simulink model "gm_DVBS"  (R2023b)
settings: Solver=FixedStepAuto  StartTime=0.0  StopTime=160000/fs  FixedStep=5e-9  RelTol=1e-3  EnableMultiTasking=on
undefined symbols (not defined in the file or in its folder): ctrlIn, fc, fs, iniStates, k, n, oneData, rb, Rcos, simDataIn, sourceData
libraries: simulink x29, hdlsllib x23, commdigbbndpm3 x4, commhdlblkcod x4, dspsrcs4 x3, whdledac x1, commsink2 x1, commcnvintrlv2 x1, commchan3 x1, dsphdlsigops2 x1, commcnvcod2 x1
(part 1 of 2)
settings Model: Creator=31651  LastModifiedBy=31651
settings SolverCC: PositivePriorityOrder=on  AutoInsertRateTranBlk=on
settings DataIOCC: ReturnWorkspaceOutputs=off
settings OptimizationCC: BlockReduction=off  ConditionallyExecuteInputs=off  DefaultUnderspecifiedDataType=single  EnhancedBackFolding=on  PassReuseOutputArgsAs=Individual arguments  ZeroExternalMemoryAtStartup=off  ZeroInternalMemoryAtStartup=off  MaxStackSize=64  OptimizeBlockOrder=speed  DifferentSizesBufferReuse=on  OptimizationCustomize=off  EfficientTunableParamExpr=on
settings DebuggingCC: ArtificialAlgebraicLoopMsg=none  InheritedTsInSrcMsg=none  SingleTaskRateTransMsg=error  ParameterPrecisionLossMsg=none  ParameterTunabilityLossMsg=error
settings HardwareCC: ProdBitPerPointer=32  ProdBitPerSizeT=32  ProdBitPerPtrDiffT=32  ProdLargestAtomicInteger=Long  ProdLargestAtomicFloat=Double  ProdWordSize=32  ProdHWDeviceType=ARM Compatible->ARM Cortex  TargetBitPerPointer=64  TargetBitPerSizeT=64  TargetBitPerPtrDiffT=64  TargetLongLongMode=on  TargetIntDivRoundTo=Zero  TargetEndianess=LittleEndian  TargetWordSize=64  TargetHWDeviceType=Custom Processor->MATLAB Host Computer  ProdEqTarget=off  HardwareBoardFeatureSet=SoCBlockset
settings ModelReferenceCC: ModelReferenceNumInstancesAllowed=Single
settings SFSimCC: MATLABDynamicMemAlloc=off
settings RTWCC: Description=Embedded Coder  SystemTargetFile=ert.tlc  HardwareBoard=ZedBoard  TLCOptions="-aInlineSetEventsForThisBaseRateFcn=TLC_FALSE -aSuppressMultiTaskScheduler=TLC_FALSE  -aRateBasedStepFcn=0"  TemplateMakefile=ert_default_tmf
settings CodeAppCC: ForceParamTrailComments=on  IgnoreCustomStorageClasses=off  OperatorAnnotations=on  SimulinkDataObjDesc=on  SFDataObjDesc=on  InsertBlockDesc=on

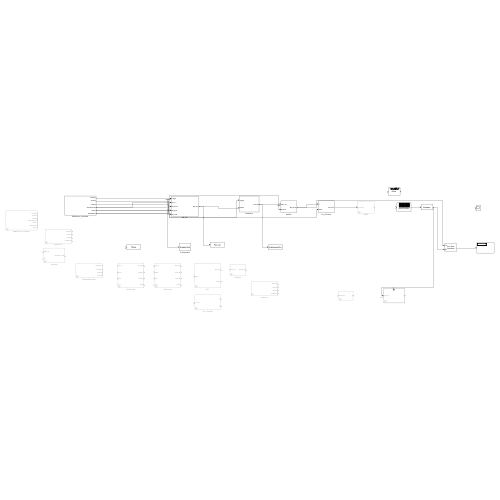
[thumbnail: Simulink's stored preview of the top-level diagram]
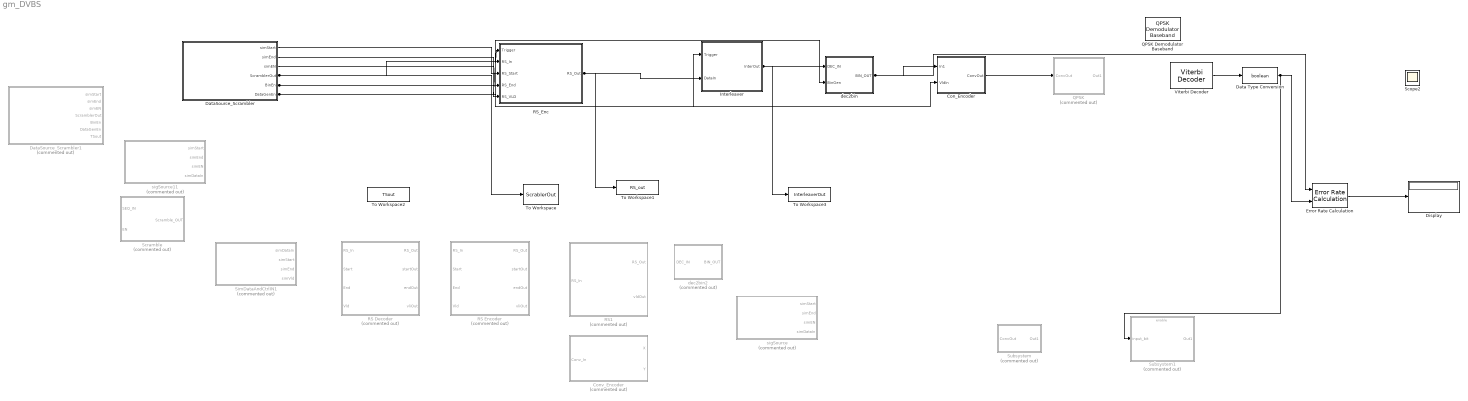
== system gm_DVBS ==
  " Scramble" : Subsystem  Commented=on
  Con_Encoder : Subsystem
  Conv_Encoder : Subsystem  Commented=on
  Data Type Conversion : DataTypeConversion  OutDataTypeStr=boolean  SaturateOnIntegerOverflow=off  RndMeth=Floor
  DataSource_Scrambler : Subsystem
  DataSource_Scrambler1 : Subsystem  Commented=on
  Display : Display
  Error Rate Calculation : commsink2/Error Rate Calculation  N=67  st_delay=0  cp_mode=Entire frame  subframe=[]  PMode=Port  WsName=ErrorVec  RsMode2=off  stop=off  numErr=100  maxBits=1e6
      settings: LibrarySourceBlock=|
      | commhdlsink/Error Rate
      | Calculation
  Interleaver : Subsystem
  QPSK : Subsystem  Commented=on
  QPSK Demodulator Baseband : commdigbbndpm3/QPSK Demodulator Baseband  OutType=Bit  DecType=Hard decision  VarSource=Dialog  Variance=1  Dec=Binary  Ph=pi/4  outDtype1=double  outDtype2=Inherit via internal rule  derotateFactorWordLen=16  derotateFactorDataTypeStr=Inherit: Same word length as input  derotateFactorLastDataTypeStr=Inherit: Same word length as input
      settings: LibrarySourceBlock=|
      | commhdldigbbndpm/QPSK
      | Demodulator
      | Baseband
  RS Decoder : Subsystem  Commented=on
  RS Encoder : Subsystem  Commented=on
  RS1 : Subsystem  Commented=on
  RS_Enc : Subsystem
  Scope2 : Scope
  SimDataAndCtrlIN1 : Subsystem  Commented=on
  Subsystem : Subsystem  Commented=on
  Subsystem1 : Subsystem  Commented=on
  To Workspace : ToWorkspace  VariableName=ScrablerOut  SampleTime=-1
      settings: Decimation=200  Save2DSignal=2-D array (concatenate along first dimension)
  To Workspace1 : ToWorkspace  VariableName=RS_out  SampleTime=-1
      settings: Decimation=200  Save2DSignal=2-D array (concatenate along first dimension)
  To Workspace2 : ToWorkspace  VariableName=TSout  SampleTime=-1
      settings: Decimation=200  Save2DSignal=2-D array (concatenate along first dimension)
  To Workspace3 : ToWorkspace  VariableName=InterleaverOut  SaveFormat=Timeseries  SampleTime=-1
  Viterbi Decoder : commcnvcod2/Viterbi Decoder  trellis=poly2trellis(7, [171 133])  isPunctured=off  punctureVector=[1; 1; 0; 1; 0; 1]  erasures=off  dectype=Hard decision  nsdecb=4  runSigValErrCheck=off  tbdepth=64  opmode=Continuous  reset=off  delayedResetAction=off  smWordLength=16  outDataType=Inherit via internal rule
  dec2bin : Subsystem
  dec2bin2 : Subsystem  Commented=on
  sigSource : Subsystem  Commented=on
  sigSource11 : Subsystem  Commented=on
  wires:
  Con_Encoder/1(ConvOut) -> QPSK/1(ConvOut)
  RS_Enc/1(RS_Out) -> Interleaver/2(DataIn), To Workspace1/1
  DataSource_Scrambler/5(BinEn) -> dec2bin/2(BinGen), Con_Encoder/2(VldIn)
  Error Rate Calculation/1 -> Display/1
  Interleaver/1(InterOut) -> dec2bin/1(DEC_IN), To Workspace3/1
  DataSource_Scrambler/6(DataGenEn) -> RS_Enc/1(Trigger), Interleaver/1(Trigger)
  DataSource_Scrambler/3(simEN) -> RS_Enc/5(RS_VLD)
  DataSource_Scrambler/2(simEnd) -> RS_Enc/4(RS_End)
  DataSource_Scrambler/1(simStart) -> RS_Enc/3(RS_Start)
  DataSource_Scrambler/4(ScramblerOut) -> To Workspace/1, RS_Enc/2(RS_In)
  dec2bin/1(BIN_OUT) -> Error Rate Calculation/1, Con_Encoder/1(In1)
  Data Type Conversion/1 -> Error Rate Calculation/2, Subsystem1/1(input_bit)
  Viterbi Decoder/1 -> Data Type Conversion/1

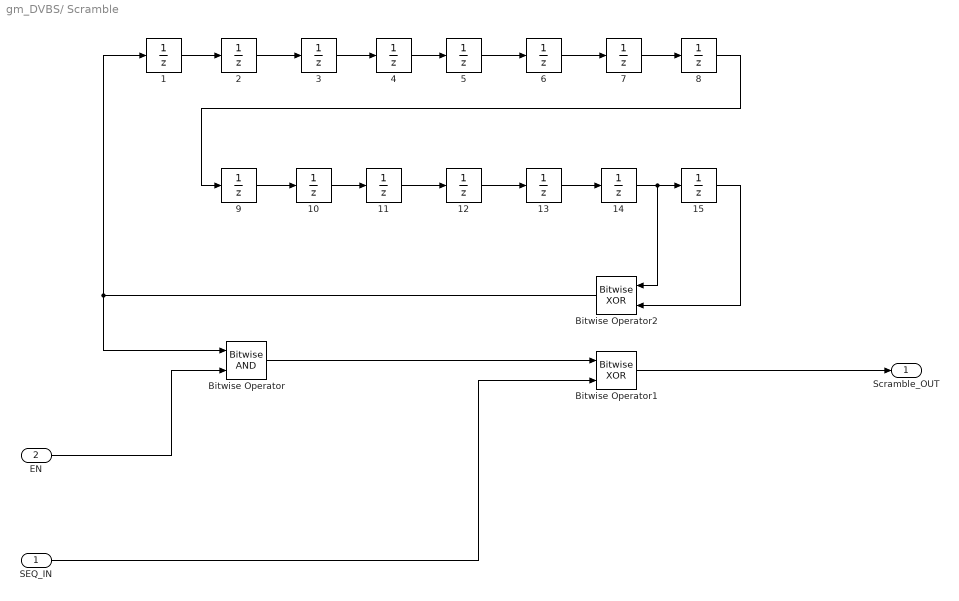
== system gm_DVBS/ Scramble ==
  SEQ_IN : Inport
  EN : Inport  Port=2  OutDataTypeStr=uint8
  1 : UnitDelay  InitialCondition=iniStates(1)  SampleTime=1/fs  HasFrameUpgradeWarning=on
  10 : UnitDelay  InitialCondition=iniStates(10)  SampleTime=-1  HasFrameUpgradeWarning=on
  11 : UnitDelay  InitialCondition=iniStates(11)  SampleTime=-1  HasFrameUpgradeWarning=on
  12 : UnitDelay  InitialCondition=iniStates(12)  SampleTime=-1  HasFrameUpgradeWarning=on
  13 : UnitDelay  InitialCondition=iniStates(13)  SampleTime=-1  HasFrameUpgradeWarning=on
  14 : UnitDelay  InitialCondition=iniStates(14)  SampleTime=-1  HasFrameUpgradeWarning=on
  15 : UnitDelay  InitialCondition=iniStates(15)  SampleTime=-1  HasFrameUpgradeWarning=on
  2 : UnitDelay  InitialCondition=iniStates(2)  SampleTime=-1  HasFrameUpgradeWarning=on
  3 : UnitDelay  InitialCondition=iniStates(3)  SampleTime=-1  HasFrameUpgradeWarning=on
  4 : UnitDelay  InitialCondition=iniStates(4)  SampleTime=-1  HasFrameUpgradeWarning=on
  5 : UnitDelay  InitialCondition=iniStates(5)  SampleTime=-1  HasFrameUpgradeWarning=on
  6 : UnitDelay  InitialCondition=iniStates(6)  SampleTime=-1  HasFrameUpgradeWarning=on
  7 : UnitDelay  InitialCondition=iniStates(7)  SampleTime=-1  HasFrameUpgradeWarning=on
  8 : UnitDelay  InitialCondition=iniStates(8)  SampleTime=-1  HasFrameUpgradeWarning=on
  9 : UnitDelay  InitialCondition=iniStates(9)  SampleTime=-1  HasFrameUpgradeWarning=on
  Bitwise Operator : simulink/Logic and Bit Operations/Bitwise Operator  logicop=AND  UseBitMask=off  NumInputPorts=2  BitMask=bin2dec('11011001')  BitMaskRealWorld=Stored Integer
      settings: LibrarySourceBlock=|
      | hdlsllib/Logic and Bit
      | Operations/Bitwise
      | Operator
  Bitwise Operator1 : simulink/Logic and Bit Operations/Bitwise Operator  logicop=XOR  UseBitMask=off  NumInputPorts=2  BitMask=bin2dec('11011001')  BitMaskRealWorld=Stored Integer
      settings: LibrarySourceBlock=|
      | hdlsllib/Logic and Bit
      | Operations/Bitwise
      | Operator
  Bitwise Operator2 : simulink/Logic and Bit Operations/Bitwise Operator  logicop=XOR  UseBitMask=off  NumInputPorts=2  BitMask=bin2dec('11011001')  BitMaskRealWorld=Stored Integer
      settings: LibrarySourceBlock=|
      | hdlsllib/Logic and Bit
      | Operations/Bitwise
      | Operator
  " Scramble_OUT" : Outport
  wires:
  Bitwise Operator1/1 -> " Scramble_OUT"/1
  SEQ_IN/1 -> Bitwise Operator1/2
  EN/1 -> Bitwise Operator/2
  Bitwise Operator/1 -> Bitwise Operator1/1
  Bitwise Operator2/1 -> 1/1, Bitwise Operator/1
  15/1 -> Bitwise Operator2/2
  12/1 -> 13/1
  13/1 -> 14/1
  14/1 -> 15/1, Bitwise Operator2/1
  6/1 -> 7/1
  7/1 -> 8/1
  11/1 -> 12/1
  8/1 -> 9/1
  10/1 -> 11/1
  9/1 -> 10/1
  1/1 -> 2/1
  3/1 -> 4/1
  2/1 -> 3/1
  4/1 -> 5/1
  5/1 -> 6/1

== system gm_DVBS/Con_Encoder ==
  In1 : Inport
  VldIn : Inport  Port=2
  Convolutional Encoder2 : whdledac/Convolutional Encoder  ConstraintLength=7  CodeGenerator=[171 133]  FeedbackConnection=0  TerminationMethod=Continuous  ResetPort=off  InitialStatePort=off  FinalStatePort=off  SimulateUsing=Code generation
  Terminator : Terminator
  ConvOut : Outport
  wires:
  VldIn/1 -> Convolutional Encoder2/2
  Convolutional Encoder2/2 -> Terminator/1
  In1/1 -> Convolutional Encoder2/1
  Convolutional Encoder2/1 -> ConvOut/1

== system gm_DVBS/Conv_Encoder ==
  Conv_In : Inport
  {0..6} (7 alike) : Delay  DelayLength=1  ShowEnablePort=on
      settings: InputPortMap=u0,e6
  Bitwise XOR : simulink/Logic and Bit Operations/Bitwise Operator  logicop=XOR  UseBitMask=off  NumInputPorts=5  BitMask=bin2dec('11011001')  BitMaskRealWorld=Stored Integer
      settings: LibrarySourceBlock=|
      | simulink/Quick Insert/Logic and Bit
      | Operations/Bitwise XOR
  Bitwise XOR1 : simulink/Logic and Bit Operations/Bitwise Operator  logicop=XOR  UseBitMask=off  NumInputPorts=5  BitMask=bin2dec('11011001')  BitMaskRealWorld=Stored Integer
      settings: LibrarySourceBlock=|
      | simulink/Quick Insert/Logic and Bit
      | Operations/Bitwise XOR
  Constant : Constant  OutDataTypeStr=boolean  SampleTime=1/rb
  int2bin : Subsystem
  int2bin1 : Subsystem
  X : Outport
  Y : Outport  Port=2
  wires:
  int2bin1/1(Out1) -> Y/1
  Bitwise XOR/1 -> int2bin/1(input)
  int2bin/1(Out1) -> X/1
  Bitwise XOR1/1 -> int2bin1/1(input)
  6/1 -> Bitwise XOR/5, Bitwise XOR1/5
  Constant/1 -> 6/2, 5/2, 4/2, 3/2, 2/2, 1/2, 0/2
  Conv_In/1 -> 0/1
  0/1 -> 1/1, Bitwise XOR/1, Bitwise XOR1/1
  1/1 -> 2/1, Bitwise XOR/2
  2/1 -> 3/1, Bitwise XOR/3, Bitwise XOR1/2
  3/1 -> 4/1, Bitwise XOR/4, Bitwise XOR1/3
  4/1 -> 5/1
  5/1 -> 6/1, Bitwise XOR1/4

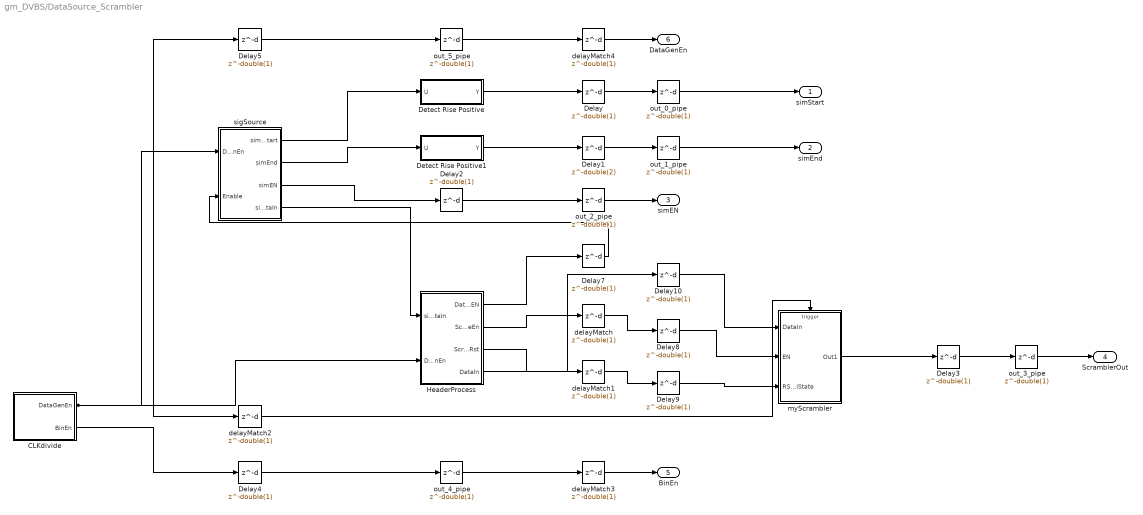
== system gm_DVBS/DataSource_Scrambler ==
  CLKdivide : Subsystem
  Delay{,2..5,7..10} (9 alike) : Delay  DelayLength=double(1)  InitialCondition=0  SampleTime=5e-09
  Delay1 : Delay  DelayLength=double(2)  InitialCondition=0  SampleTime=5e-09
  Detect Rise Positive : Subsystem  mask(Detect Rise Positive){vinit=double(0), InputProcessing=Elements as channels (sample based), OutDataTypeStr=boolean}
      mask prompts: vinit "Simulink:masks:InitialCondition_MP"; InputProcessing "Simulink:masks:InputProcessing_MP"; OutDataTypeStr "Simulink:masks:OutputDataType_MP"
      mask help: Simulink:masks:DetectRisePositive_MD
      mask init:
      | InputProcessing = 'Elements as channels (sample based)';
      | OutDataTypeStr = 'boolean';
      | vinit = double(0);
      mask TypeOptions InputProcessing: Simulink:masks:ColumnsAsChannelsFrameBased | Simulink:masks:ElementsAsChannelsSampleBased
      mask TypeOptions OutDataTypeStr: Simulink:masks:uint8 | Simulink:masks:boolean
      mask Display: fprintf('U > 0\n&  NOT\nU/z > 0')
  Detect Rise Positive1 : Subsystem  mask(Detect Rise Positive){vinit=double(0), InputProcessing=Elements as channels (sample based), OutDataTypeStr=boolean}
      mask prompts: vinit "Simulink:masks:InitialCondition_MP"; InputProcessing "Simulink:masks:InputProcessing_MP"; OutDataTypeStr "Simulink:masks:OutputDataType_MP"
      mask help: Simulink:masks:DetectRisePositive_MD
      mask init:
      | InputProcessing = 'Elements as channels (sample based)';
      | OutDataTypeStr = 'boolean';
      | vinit = double(0);
      mask TypeOptions InputProcessing: Simulink:masks:ColumnsAsChannelsFrameBased | Simulink:masks:ElementsAsChannelsSampleBased
      mask TypeOptions OutDataTypeStr: Simulink:masks:uint8 | Simulink:masks:boolean
      mask Display: fprintf('U > 0\n&  NOT\nU/z > 0')
  HeaderProcess : Subsystem
  delayMatch{,1..4} (5 alike) : Delay  DelayLength=double(1)  InitialCondition=0  SampleTime=5e-09
  myScrambler : Subsystem
  out_0_pipe : Delay  DelayLength=double(1)  InitialCondition=0  SampleTime=5e-09
  out_1_pipe : Delay  DelayLength=double(1)  InitialCondition=0  SampleTime=5e-09
  out_2_pipe : Delay  DelayLength=double(1)  InitialCondition=0  SampleTime=5e-09
  out_3_pipe : Delay  DelayLength=double(1)  InitialCondition=0  SampleTime=5e-09
  out_4_pipe : Delay  DelayLength=double(1)  InitialCondition=0  SampleTime=5e-09
  out_5_pipe : Delay  DelayLength=double(1)  InitialCondition=0  SampleTime=5e-09
  sigSource : Subsystem
  simStart : Outport  SampleTime=5e-09
  simEnd : Outport  Port=2  SampleTime=5e-09
  simEN : Outport  Port=3  SampleTime=5e-09
  ScramblerOut : Outport  Port=4  SampleTime=5e-09
  BinEn : Outport  Port=5  SampleTime=5e-09  VectorParamsAs1DForOutWhenUnconnected=off
  DataGenEn : Outport  Port=6  SampleTime=5e-09  VectorParamsAs1DForOutWhenUnconnected=off
  wires:
  delayMatch2/1 -> myScrambler/Trigger
  CLKdivide/2(BinEn) -> Delay4/1
  Delay/1 -> out_0_pipe/1
  Delay1/1 -> out_1_pipe/1
  Delay10/1 -> myScrambler/1(DataIn)
  Delay2/1 -> out_2_pipe/1
  Delay3/1 -> out_3_pipe/1
  Delay4/1 -> out_4_pipe/1
  Delay5/1 -> out_5_pipe/1
  Delay8/1 -> myScrambler/2(EN)
  Delay9/1 -> myScrambler/3(RST_IniState)
  Detect Rise Positive/1(Y) -> Delay/1
  Detect Rise Positive1/1(Y) -> Delay1/1
  myScrambler/1(Out1) -> Delay3/1
  out_0_pipe/1 -> simStart/1
  out_1_pipe/1 -> simEnd/1
  out_2_pipe/1 -> simEN/1
  out_3_pipe/1 -> ScramblerOut/1
  delayMatch3/1 -> BinEn/1
  delayMatch4/1 -> DataGenEn/1
  CLKdivide/1(DataGenEn) -> delayMatch2/1, Delay5/1, sigSource/1(DataGenEn), HeaderProcess/2(DataGenEn)
  out_4_pipe/1 -> delayMatch3/1
  out_5_pipe/1 -> delayMatch4/1
  delayMatch/1 -> Delay8/1
  delayMatch1/1 -> Delay9/1
  HeaderProcess/1(DataGenEN) -> Delay7/1
  sigSource/1(simStart) -> Detect Rise Positive/1(U)
  sigSource/2(simEnd) -> Detect Rise Positive1/1(U)
  sigSource/3(simEN) -> Delay2/1
  Delay7/1 -> sigSource/2(Enable)
  HeaderProcess/2(ScrambleEn) -> delayMatch/1
  HeaderProcess/3(ScrambleRst) -> delayMatch1/1
  HeaderProcess/4(DataIn) -> Delay10/1
  sigSource/4(simDataIn) -> HeaderProcess/1(simDataIn)

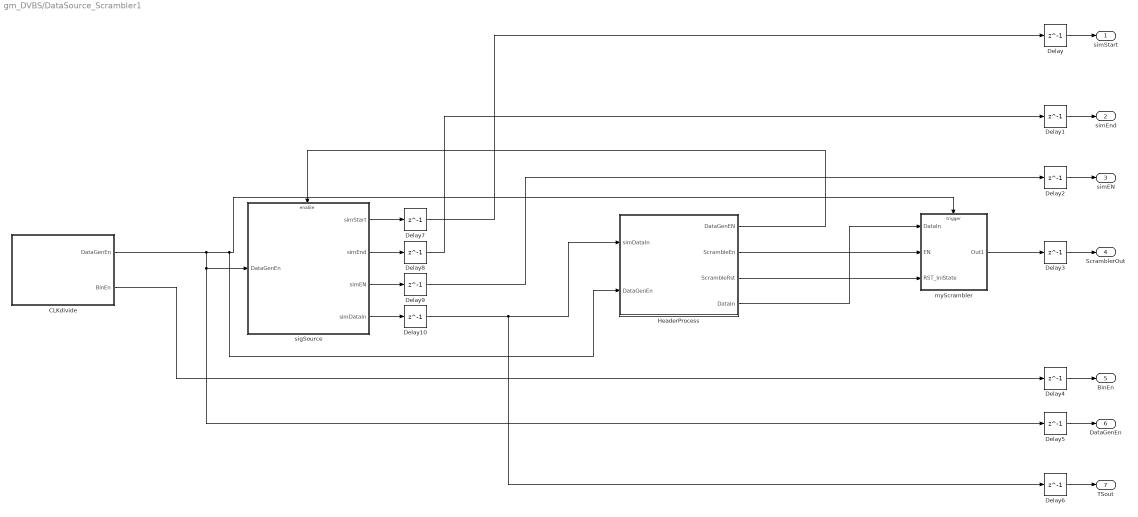
== system gm_DVBS/DataSource_Scrambler1 ==
  CLKdivide : Subsystem
  Delay{,1..10} (11 alike) : Delay  DelayLength=1
  HeaderProcess : Subsystem
  myScrambler : Subsystem
  sigSource : Subsystem
  simStart : Outport
  simEnd : Outport  Port=2
  simEN : Outport  Port=3
  ScramblerOut : Outport  Port=4
  BinEn : Outport  Port=5  VectorParamsAs1DForOutWhenUnconnected=off
  DataGenEn : Outport  Port=6  VectorParamsAs1DForOutWhenUnconnected=off
  TSout : Outport  Port=7  VectorParamsAs1DForOutWhenUnconnected=off
  wires:
  Delay10/1 -> Delay6/1, HeaderProcess/1(simDataIn)
  Delay9/1 -> Delay2/1
  Delay8/1 -> Delay1/1
  Delay7/1 -> Delay/1
  HeaderProcess/4(DataIn) -> myScrambler/1(DataIn)
  HeaderProcess/3(ScrambleRst) -> myScrambler/3(RST_IniState)
  HeaderProcess/2(ScrambleEn) -> myScrambler/2(EN)
  HeaderProcess/1(DataGenEN) -> sigSource/Enable
  Delay6/1 -> TSout/1
  Delay5/1 -> DataGenEn/1
  Delay4/1 -> BinEn/1
  Delay3/1 -> ScramblerOut/1
  Delay2/1 -> simEN/1
  Delay1/1 -> simEnd/1
  Delay/1 -> simStart/1
  CLKdivide/2(BinEn) -> Delay4/1
  CLKdivide/1(DataGenEn) -> sigSource/1(DataGenEn), Delay5/1, HeaderProcess/2(DataGenEn), myScrambler/Trigger
  sigSource/4(simDataIn) -> Delay10/1
  sigSource/2(simEnd) -> Delay8/1
  myScrambler/1(Out1) -> Delay3/1
  sigSource/1(simStart) -> Delay7/1
  sigSource/3(simEN) -> Delay9/1

== system gm_DVBS/Interleaver ==
  Trigger : Inport
  DataIn : Inport  Port=2
  Con_Interleaver : Subsystem
  InterOut : Outport
  wires:
  DataIn/1 -> Con_Interleaver/1(In1)
  Con_Interleaver/1(Out1) -> InterOut/1
  Trigger/1 -> Con_Interleaver/Trigger

== system gm_DVBS/QPSK ==
  ConvOut : Inport
  AWGN Channel : commchan3/AWGN Channel  LegacyMode=off  NoiseMethod="Signal to noise ratio  (SNR)"  noiseMode="Signal to noise ratio  (SNR)"  EbNo=10  EsNo=10  SNR=10  BitsPerSymbol=1  SignalPower=1  SamplesPerSymbol=1  SymbolPeriod=1  VarianceSource=Parameter  Variance=1  RandomStream=Global stream  Seed=67  SimulateUsing=Code generation
  Buffer : Buffer  N=208*8  OutputFrames=off
  Buffer1 : Buffer  N=208*8  OutputFrames=off
  Constellation Diagram : ConstellationDiagram  WindowPosition=[382.000000,84.000000,600.000000,600.000000,]  ScopeFrameLocation=window
  Constellation Diagram1 : ConstellationDiagram  WindowPosition=[382.000000,84.000000,600.000000,600.000000,]  ScopeFrameLocation=window
  QPSK_Modulation : Subsystem
  Spectrum Analyzer : SpectrumAnalyzer  WindowPosition=[560.000000,290.000000,800.000000,500.000000,]  ScopeFrameLocation=window  Span=200000000  StartFrequency=-100000000  StopFrequency=100000000  YLimits=[-144.86209113,49.80146436]
  Spectrum Analyzer1 : SpectrumAnalyzer  WindowPosition=[560.000000,290.000000,800.000000,500.000000,]  ScopeFrameLocation=window  Span=200000000  StartFrequency=-100000000  StopFrequency=100000000  YLimits=[-22.12674688,36.16849279]
  Subsystem : Subsystem
  Out1 : Outport
  wires:
  Buffer1/1 -> Constellation Diagram1/1
  QPSK_Modulation/2(Out2) -> Buffer/1
  Buffer/1 -> Constellation Diagram/1
  AWGN Channel/1 -> Subsystem/1(In1), Buffer1/1, Spectrum Analyzer1/1
  ConvOut/1 -> QPSK_Modulation/1(In1)
  QPSK_Modulation/1(Out1) -> Spectrum Analyzer/1, AWGN Channel/1

== system gm_DVBS/RS Decoder ==
  RS_In : Inport  OutDataTypeStr=uint8
  Start : Inport  Port=2
  End : Inport  Port=3
  Vld : Inport  Port=4
  Data Type Conversion : DataTypeConversion  OutDataTypeStr=boolean  SaturateOnIntegerOverflow=off  RndMeth=Floor
  Data Type Conversion1 : DataTypeConversion  OutDataTypeStr=boolean  SaturateOnIntegerOverflow=off  RndMeth=Floor
  Data Type Conversion2 : DataTypeConversion  OutDataTypeStr=boolean  SaturateOnIntegerOverflow=off  RndMeth=Floor
  Integer-Output RS Decoder HDL Optimized : commhdlblkcod/Integer-Output RS Decoder HDL Optimized  CodewordLength=n  MessageLength=k  PrimitivePolynomialSource=Property  PrimitivePolynomial=[1 0 0 0 1 1 1 0 1]  BSource=Property  B=0  NumErrorsOutputPort=off  SimulateUsing=Code generation
  Terminator : Terminator
  RS_Out : Outport  OutDataTypeStr=uint8
  startOut : Outport  Port=2
  endOut : Outport  Port=3
  vliOut : Outport  Port=4
  wires:
  Integer-Output RS Decoder HDL Optimized/5 -> Terminator/1
  Integer-Output RS Decoder HDL Optimized/4 -> vliOut/1
  Integer-Output RS Decoder HDL Optimized/3 -> endOut/1
  Integer-Output RS Decoder HDL Optimized/2 -> startOut/1
  Vld/1 -> Data Type Conversion2/1
  End/1 -> Data Type Conversion1/1
  Start/1 -> Data Type Conversion/1
  Integer-Output RS Decoder HDL Optimized/1 -> RS_Out/1
  RS_In/1 -> Integer-Output RS Decoder HDL Optimized/1
  Data Type Conversion2/1 -> Integer-Output RS Decoder HDL Optimized/4
  Data Type Conversion1/1 -> Integer-Output RS Decoder HDL Optimized/3
  Data Type Conversion/1 -> Integer-Output RS Decoder HDL Optimized/2

== system gm_DVBS/RS Encoder ==
  RS_In : Inport  OutDataTypeStr=uint8
  Start : Inport  Port=2
  End : Inport  Port=3
  Vld : Inport  Port=4
  Data Type Conversion : DataTypeConversion  OutDataTypeStr=boolean  SaturateOnIntegerOverflow=off  RndMeth=Floor
  Data Type Conversion1 : DataTypeConversion  OutDataTypeStr=boolean  SaturateOnIntegerOverflow=off  RndMeth=Floor
  Data Type Conversion2 : DataTypeConversion  OutDataTypeStr=boolean  SaturateOnIntegerOverflow=off  RndMeth=Floor
  Integer-Input RS Encoder HDL Optimized : commhdlblkcod/Integer-Input RS Encoder HDL Optimized  CodewordLength=n  MessageLength=k  PrimitivePolynomialSource=Property  PrimitivePolynomial=[1 0 0 0 1 1 1 0 1]  PuncturePatternSource=None  PuncturePattern=[ ones( 2, 1 ); zeros( 2, 1 ) ]  BSource=Property  B=0  SimulateUsing=Code generation
  RS_Out : Outport  OutDataTypeStr=uint8
  startOut : Outport  Port=2
  endOut : Outport  Port=3
  vliOut : Outport  Port=4
  wires:
  Integer-Input RS Encoder HDL Optimized/4 -> vliOut/1
  Integer-Input RS Encoder HDL Optimized/3 -> endOut/1
  Integer-Input RS Encoder HDL Optimized/2 -> startOut/1
  Vld/1 -> Data Type Conversion2/1
  End/1 -> Data Type Conversion1/1
  Start/1 -> Data Type Conversion/1
  Integer-Input RS Encoder HDL Optimized/1 -> RS_Out/1
  RS_In/1 -> Integer-Input RS Encoder HDL Optimized/1
  Data Type Conversion2/1 -> Integer-Input RS Encoder HDL Optimized/4
  Data Type Conversion1/1 -> Integer-Input RS Encoder HDL Optimized/3
  Data Type Conversion/1 -> Integer-Input RS Encoder HDL Optimized/2

== system gm_DVBS/RS1 ==
  RS_In : Inport  OutDataTypeStr=uint8
  Data Type Conversion : DataTypeConversion  OutDataTypeStr=boolean  SaturateOnIntegerOverflow=off  RndMeth=Floor
  Data Type Conversion1 : DataTypeConversion  OutDataTypeStr=boolean  SaturateOnIntegerOverflow=off  RndMeth=Floor
  Data Type Conversion2 : DataTypeConversion  OutDataTypeStr=boolean  SaturateOnIntegerOverflow=off  RndMeth=Floor
  Integer-Input RS Encoder HDL Optimized : commhdlblkcod/Integer-Input RS Encoder HDL Optimized  CodewordLength=n  MessageLength=k  PrimitivePolynomialSource=Property  PrimitivePolynomial=[1 0 0 0 1 1 1 0 1]  PuncturePatternSource=None  PuncturePattern=[ ones( 2, 1 ); zeros( 2, 1 ) ]  BSource=Property  B=0  SimulateUsing=Code generation
  Signal From Workspace1 : dspsrcs4/Signal From Workspace  X=simStart  Ts=1/rb  nsamps=1  OutputAfterFinalValue=Setting to zero  ignoreOrWarnInputAndFrameLengths=off  OutputFrames=off
  Signal From Workspace2 : dspsrcs4/Signal From Workspace  X=simEnd  Ts=1/rb  nsamps=1  OutputAfterFinalValue=Setting to zero  ignoreOrWarnInputAndFrameLengths=off  OutputFrames=off
  Signal From Workspace3 : dspsrcs4/Signal From Workspace  X=simValidIn  Ts=1/rb  nsamps=1  OutputAfterFinalValue=Setting to zero  ignoreOrWarnInputAndFrameLengths=off  OutputFrames=off
  RS_Out : Outport  OutDataTypeStr=uint8
  vldOut : Outport  Port=2  OutDataTypeStr=boolean
  wires:
  Integer-Input RS Encoder HDL Optimized/4 -> vldOut/1
  Integer-Input RS Encoder HDL Optimized/1 -> RS_Out/1
  RS_In/1 -> Integer-Input RS Encoder HDL Optimized/1
  Data Type Conversion2/1 -> Integer-Input RS Encoder HDL Optimized/4
  Signal From Workspace1/1 -> Data Type Conversion/1
  Signal From Workspace2/1 -> Data Type Conversion1/1
  Signal From Workspace3/1 -> Data Type Conversion2/1
  Data Type Conversion1/1 -> Integer-Input RS Encoder HDL Optimized/3
  Data Type Conversion/1 -> Integer-Input RS Encoder HDL Optimized/2

== system gm_DVBS/RS_Enc ==
  Trigger : Inport  OutDataTypeStr=boolean
  RS_In : Inport  Port=2
  RS_Start : Inport  Port=3
  RS_End : Inport  Port=4
  RS_VLD : Inport  Port=5
  RS : Subsystem
  RS_Out : Outport
  wires:
  Trigger/1 -> RS/Trigger
  RS_Start/1 -> RS/2(RS_Start)
  RS_VLD/1 -> RS/4(RS_VLD)
  RS_End/1 -> RS/3(RS_End)
  RS_In/1 -> RS/1(RS_In)
  RS/1(RS_Out) -> RS_Out/1

== system gm_DVBS/SimDataAndCtrlIN1 ==
  1-D Lookup Table : Lookup_n-D  NumberOfTableDimensions=1  LookupTableObject=''  BreakpointsForDimension1=[0:187]  BreakpointsForDimension1FirstPoint=10  BreakpointsForDimension2FirstPoint=10  BreakpointsForDimension1Spacing=12  BreakpointsForDimension2Spacing=12  IndexSearchMethod=Evenly spaced points  Table=simDataIn  InterpMethod=Flat  DiagnosticForOutOfRangeInput=Error  InternalRulePriority=Speed  OutDataTypeStr=uint8  RndMeth=Simplest
  1-D Lookup Table1 : Lookup_n-D  NumberOfTableDimensions=1  LookupTableObject=''  BreakpointsForDimension1=[0:203]  BreakpointsForDimension1FirstPoint=10  BreakpointsForDimension2FirstPoint=10  BreakpointsForDimension1Spacing=12  BreakpointsForDimension2Spacing=12  IndexSearchMethod=Evenly spaced points  Table=uint8(ctrlIn(:,1))'  InterpMethod=Flat  DiagnosticForOutOfRangeInput=Error  InternalRulePriority=Speed  OutDataTypeStr=uint8  RndMeth=Simplest
  1-D Lookup Table2 : Lookup_n-D  NumberOfTableDimensions=1  LookupTableObject=''  BreakpointsForDimension1=[0:203]  BreakpointsForDimension1FirstPoint=10  BreakpointsForDimension2FirstPoint=10  BreakpointsForDimension1Spacing=12  BreakpointsForDimension2Spacing=12  IndexSearchMethod=Evenly spaced points  Table=uint8(ctrlIn(:,2))'  InterpMethod=Flat  DiagnosticForOutOfRangeInput=Error  InternalRulePriority=Speed  OutDataTypeStr=uint8  RndMeth=Simplest
  1-D Lookup Table3 : Lookup_n-D  NumberOfTableDimensions=1  LookupTableObject=''  BreakpointsForDimension1=[0:203]  BreakpointsForDimension1FirstPoint=10  BreakpointsForDimension2FirstPoint=10  BreakpointsForDimension1Spacing=12  BreakpointsForDimension2Spacing=12  IndexSearchMethod=Evenly spaced points  Table=uint8(ctrlIn(:,3))'  InterpMethod=Flat  DiagnosticForOutOfRangeInput=Error  InternalRulePriority=Speed  OutDataTypeStr=uint8  RndMeth=Simplest
  DATA_IN : DataTypeConversion  OutDataTypeStr=inDataType  SaturateOnIntegerOverflow=off  RndMeth=Floor
  DATA_IN1 : DataTypeConversion  OutDataTypeStr=boolean  SaturateOnIntegerOverflow=off  RndMeth=Floor
  DATA_IN2 : DataTypeConversion  OutDataTypeStr=boolean  SaturateOnIntegerOverflow=off  RndMeth=Floor
  DATA_IN3 : DataTypeConversion  OutDataTypeStr=boolean  SaturateOnIntegerOverflow=off  RndMeth=Floor
  HDL Counter : hdlsllib/Sources/HDL Counter  CountType=Count limited  CountInit=0  CountStep=1  CountMax=k-1  CountFromType=Initial value  CountFrom=0  CountResetPort=off  CountLoadPort=off  CountEnbPort=off  CountDirPort=off  CountHitOutputPort=off  CountDataType=Unsigned  CountWordLen=8  CountFracLen=0  CountSampTime=1/fs
  simDataIn : Outport
  simStart : Outport  Port=2  OutDataTypeStr=boolean
  simEnd : Outport  Port=3  OutDataTypeStr=boolean
  simVld : Outport  Port=4  OutDataTypeStr=boolean
  wires:
  DATA_IN3/1 -> simVld/1
  DATA_IN2/1 -> simEnd/1
  DATA_IN1/1 -> simStart/1
  1-D Lookup Table3/1 -> DATA_IN3/1
  1-D Lookup Table2/1 -> DATA_IN2/1
  1-D Lookup Table1/1 -> DATA_IN1/1
  DATA_IN/1 -> simDataIn/1
  HDL Counter/1 -> 1-D Lookup Table/1, 1-D Lookup Table1/1, 1-D Lookup Table2/1, 1-D Lookup Table3/1
  1-D Lookup Table/1 -> DATA_IN/1

== system gm_DVBS/Subsystem ==
  note: I路
  note: Q路
  ConvOut : Inport
  Add : Sum
  Complex to Real-Imag : ComplexToRealImag
  Product : Product
  Product1 : Product
  QPSK Modulator Baseband : commdigbbndpm3/QPSK Modulator Baseband  InType=Bit  Enc=Gray  Ph=pi/4  outDtype=double  outWordLen=16  outUDDataType=sfix(16)  outFracLenMode=Best precision  outFracLen=15  outDataTypeStr=double  outLastDataTypeStr=double
      settings: LibrarySourceBlock=|
      | commhdldigbbndpm/QPSK
      | Modulator
      | Baseband
  RT : RateTransition  OutPortSampleTime=2.5e-06
  RT1 : RateTransition  OutPortSampleTime=2.5e-06
  Scope : Scope
  Scope1 : Scope
  Sign : Signum
  Sign1 : Signum
  Subsystem : Subsystem
  Zero-Order Hold1 : ZeroOrderHold  SampleTime=1/fs
  Out1 : Outport
  wires:
  RT1/1 -> Add/2
  RT/1 -> Product/2
  Product1/1 -> RT1/1
  Sign/1 -> Product/1
  Subsystem/2(cos) -> RT/1
  Zero-Order Hold1/1 -> Product1/2
  Add/1 -> Out1/1, Scope1/1
  Product/1 -> Scope/1, Add/1
  Subsystem/1(sin) -> Product1/1
  Sign1/1 -> Zero-Order Hold1/1
  Complex to Real-Imag/2 -> Sign1/1
  QPSK Modulator Baseband/1 -> Complex to Real-Imag/1
  Complex to Real-Imag/1 -> Sign/1
  ConvOut/1 -> QPSK Modulator Baseband/1

== system gm_DVBS/Subsystem1 ==
  input_bit : Inport  OutDataTypeStr=uint8
  Enable : EnablePort
  Bits to Word : hdlsllib/Logic and Bit Operations/Bits to Word
  Buffer : Buffer  N=8  OutputFrames=off
  Data Type Conversion : DataTypeConversion  OutMax=1  OutDataTypeStr=fixdt(0,1,0)  SaturateOnIntegerOverflow=off  RndMeth=Floor
  Out1 : Outport
  wires:
  Data Type Conversion/1 -> Bits to Word/1
  Bits to Word/1 -> Out1/1
  Buffer/1 -> Data Type Conversion/1
  input_bit/1 -> Buffer/1

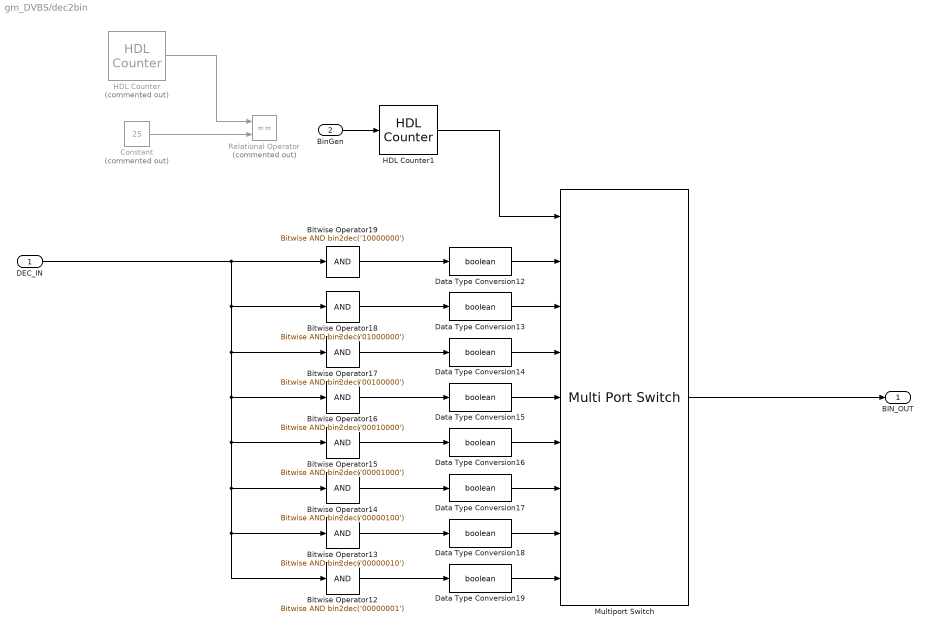
== system gm_DVBS/dec2bin ==
  DEC_IN : Inport  OutDataTypeStr=uint8
  BinGen : Inport  Port=2
  Bitwise Operator12 : simulink/Logic and Bit Operations/Bitwise Operator  logicop=AND  UseBitMask=on  BitMask=bin2dec('00000001')  BitMaskRealWorld=Stored Integer
  Bitwise Operator13 : simulink/Logic and Bit Operations/Bitwise Operator  logicop=AND  UseBitMask=on  BitMask=bin2dec('00000010')  BitMaskRealWorld=Stored Integer
  Bitwise Operator14 : simulink/Logic and Bit Operations/Bitwise Operator  logicop=AND  UseBitMask=on  BitMask=bin2dec('00000100')  BitMaskRealWorld=Stored Integer
  Bitwise Operator15 : simulink/Logic and Bit Operations/Bitwise Operator  logicop=AND  UseBitMask=on  BitMask=bin2dec('00001000')  BitMaskRealWorld=Stored Integer
  Bitwise Operator16 : simulink/Logic and Bit Operations/Bitwise Operator  logicop=AND  UseBitMask=on  BitMask=bin2dec('00010000')  BitMaskRealWorld=Stored Integer
  Bitwise Operator17 : simulink/Logic and Bit Operations/Bitwise Operator  logicop=AND  UseBitMask=on  BitMask=bin2dec('00100000')  BitMaskRealWorld=Stored Integer
  Bitwise Operator18 : simulink/Logic and Bit Operations/Bitwise Operator  logicop=AND  UseBitMask=on  BitMask=bin2dec('01000000')  BitMaskRealWorld=Stored Integer
  Bitwise Operator19 : simulink/Logic and Bit Operations/Bitwise Operator  logicop=AND  UseBitMask=on  BitMask=bin2dec('10000000')  BitMaskRealWorld=Stored Integer
  Constant : Constant  Commented=on  Value=25  OutDataTypeStr=uint8
  Data Type Conversion{12..19} (8 alike) : DataTypeConversion  OutDataTypeStr=boolean  SaturateOnIntegerOverflow=off  RndMeth=Floor
  HDL Counter : hdlsllib/Sources/HDL Counter  Commented=on  CountType=Count limited  CountInit=1  CountStep=1  CountMax=25  CountFromType=Initial value  CountFrom=1  CountResetPort=off  CountLoadPort=off  CountEnbPort=off  CountDirPort=off  CountHitOutputPort=off  CountDataType=Unsigned  CountWordLen=8  CountFracLen=0  CountSampTime=1/fs
  HDL Counter1 : hdlsllib/Sources/HDL Counter  CountType=Count limited  CountInit=1  CountStep=1  CountMax=8  CountFromType=Specify  CountFrom=1  CountResetPort=off  CountLoadPort=off  CountEnbPort=on  CountDirPort=off  CountHitOutputPort=off  CountDataType=Unsigned  CountWordLen=8  CountFracLen=0  CountSampTime=1/fs
  Multiport Switch : MultiPortSwitch  Inputs=8  DiagnosticForDefault=Warning  SaturateOnIntegerOverflow=off  InputSameDT=off
  Relational Operator : RelationalOperator  Commented=on  Operator===  OutDataTypeStr=boolean  RndMeth=Simplest  InputSameDT=off
  BIN_OUT : Outport
  wires:
  HDL Counter1/1 -> Multiport Switch/1
  BinGen/1 -> HDL Counter1/1
  Constant/1 -> Relational Operator/2
  HDL Counter/1 -> Relational Operator/1
  Multiport Switch/1 -> BIN_OUT/1
  DEC_IN/1 -> Bitwise Operator17/1, Bitwise Operator14/1, Bitwise Operator12/1, Bitwise Operator13/1, Bitwise Operator15/1, Bitwise Operator16/1, Bitwise Operator18/1, Bitwise Operator19/1
  Bitwise Operator17/1 -> Data Type Conversion14/1
  Data Type Conversion19/1 -> Multiport Switch/9
  Data Type Conversion17/1 -> Multiport Switch/7
  Data Type Conversion13/1 -> Multiport Switch/3
  Bitwise Operator12/1 -> Data Type Conversion19/1
  Data Type Conversion16/1 -> Multiport Switch/6
  Data Type Conversion15/1 -> Multiport Switch/5
  Data Type Conversion14/1 -> Multiport Switch/4
  Data Type Conversion18/1 -> Multiport Switch/8
  Data Type Conversion12/1 -> Multiport Switch/2
  Bitwise Operator16/1 -> Data Type Conversion15/1
  Bitwise Operator14/1 -> Data Type Conversion17/1
  Bitwise Operator15/1 -> Data Type Conversion16/1
  Bitwise Operator19/1 -> Data Type Conversion12/1
  Bitwise Operator18/1 -> Data Type Conversion13/1
  Bitwise Operator13/1 -> Data Type Conversion18/1

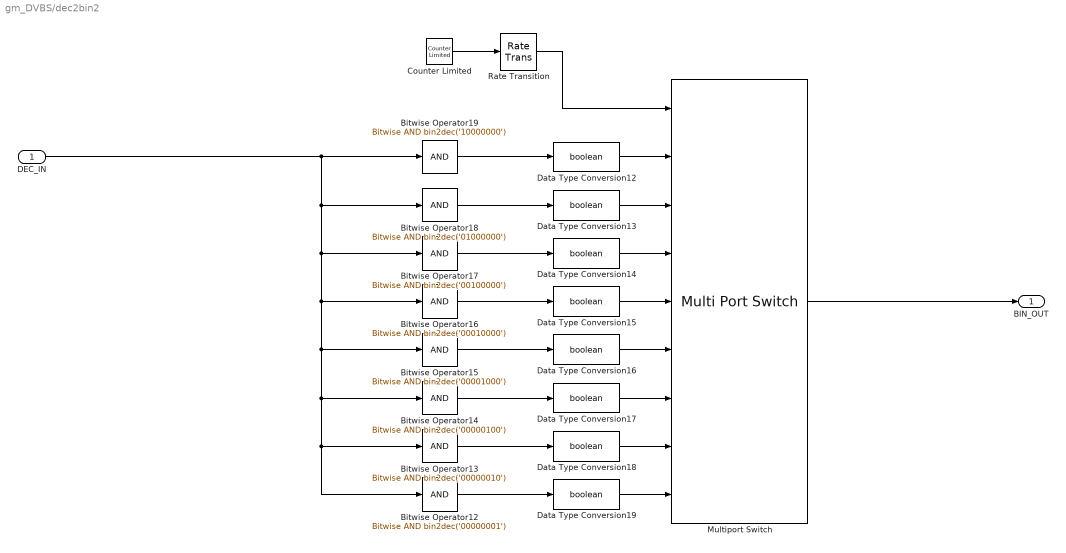
== system gm_DVBS/dec2bin2 ==
  DEC_IN : Inport  OutDataTypeStr=uint8
  Bitwise Operator12 : simulink/Logic and Bit Operations/Bitwise Operator  logicop=AND  UseBitMask=on  BitMask=bin2dec('00000001')  BitMaskRealWorld=Stored Integer
  Bitwise Operator13 : simulink/Logic and Bit Operations/Bitwise Operator  logicop=AND  UseBitMask=on  BitMask=bin2dec('00000010')  BitMaskRealWorld=Stored Integer
  Bitwise Operator14 : simulink/Logic and Bit Operations/Bitwise Operator  logicop=AND  UseBitMask=on  BitMask=bin2dec('00000100')  BitMaskRealWorld=Stored Integer
  Bitwise Operator15 : simulink/Logic and Bit Operations/Bitwise Operator  logicop=AND  UseBitMask=on  BitMask=bin2dec('00001000')  BitMaskRealWorld=Stored Integer
  Bitwise Operator16 : simulink/Logic and Bit Operations/Bitwise Operator  logicop=AND  UseBitMask=on  BitMask=bin2dec('00010000')  BitMaskRealWorld=Stored Integer
  Bitwise Operator17 : simulink/Logic and Bit Operations/Bitwise Operator  logicop=AND  UseBitMask=on  BitMask=bin2dec('00100000')  BitMaskRealWorld=Stored Integer
  Bitwise Operator18 : simulink/Logic and Bit Operations/Bitwise Operator  logicop=AND  UseBitMask=on  BitMask=bin2dec('01000000')  BitMaskRealWorld=Stored Integer
  Bitwise Operator19 : simulink/Logic and Bit Operations/Bitwise Operator  logicop=AND  UseBitMask=on  BitMask=bin2dec('10000000')  BitMaskRealWorld=Stored Integer
  Counter Limited : hdlsllib/Sources/Counter Limited  uplimit=7  tsamp=0.125/rb
  Data Type Conversion{12..19} (8 alike) : DataTypeConversion  OutDataTypeStr=boolean  SaturateOnIntegerOverflow=off  RndMeth=Floor
  Multiport Switch : MultiPortSwitch  DataPortOrder=Zero-based contiguous  Inputs=8  zeroidx=on  SaturateOnIntegerOverflow=off  InputSameDT=off
  Rate Transition : RateTransition  OutPortSampleTime=0.125/rb
  BIN_OUT : Outport
  wires:
  Rate Transition/1 -> Multiport Switch/1
  DEC_IN/1 -> Bitwise Operator19/1, Bitwise Operator17/1, Bitwise Operator14/1, Bitwise Operator12/1, Bitwise Operator13/1, Bitwise Operator15/1, Bitwise Operator16/1, Bitwise Operator18/1
  Counter Limited/1 -> Rate Transition/1
  Multiport Switch/1 -> BIN_OUT/1
  Bitwise Operator17/1 -> Data Type Conversion14/1
  Data Type Conversion19/1 -> Multiport Switch/9
  Data Type Conversion17/1 -> Multiport Switch/7
  Data Type Conversion13/1 -> Multiport Switch/3
  Bitwise Operator12/1 -> Data Type Conversion19/1
  Data Type Conversion16/1 -> Multiport Switch/6
  Data Type Conversion15/1 -> Multiport Switch/5
  Data Type Conversion14/1 -> Multiport Switch/4
  Data Type Conversion18/1 -> Multiport Switch/8
  Data Type Conversion12/1 -> Multiport Switch/2
  Bitwise Operator16/1 -> Data Type Conversion15/1
  Bitwise Operator14/1 -> Data Type Conversion17/1
  Bitwise Operator15/1 -> Data Type Conversion16/1
  Bitwise Operator19/1 -> Data Type Conversion12/1
  Bitwise Operator18/1 -> Data Type Conversion13/1
  Bitwise Operator13/1 -> Data Type Conversion18/1

== system gm_DVBS/sigSource ==
  1-D Lookup Table : Lookup_n-D  NumberOfTableDimensions=1  LookupTableObject=''  BreakpointsForDimension1=[0:18800-1]'  BreakpointsForDimension1FirstPoint=10  BreakpointsForDimension2FirstPoint=10  BreakpointsForDimension1Spacing=12  BreakpointsForDimension2Spacing=12  IndexSearchMethod=Evenly spaced points  Table=sourceData  InterpMethod=Flat  DiagnosticForOutOfRangeInput=Error  InternalRulePriority=Speed  OutDataTypeStr=uint8  RndMeth=Simplest
  1-D Lookup Table1 : Lookup_n-D  NumberOfTableDimensions=1  LookupTableObject=''  BreakpointsForDimension1=[0:1020-1]'  BreakpointsForDimension1FirstPoint=10  BreakpointsForDimension2FirstPoint=10  BreakpointsForDimension1Spacing=12  BreakpointsForDimension2Spacing=12  IndexSearchMethod=Evenly spaced points  Table=oneData  InterpMethod=Flat  DiagnosticForOutOfRangeInput=Error  InternalRulePriority=Speed  OutDataTypeStr=uint8  RndMeth=Simplest
  Constant : Constant  Value=204  OutDataTypeStr=uint16  SampleTime=1/fs
  DATA_IN : DataTypeConversion  OutDataTypeStr=inDataType  SaturateOnIntegerOverflow=off  RndMeth=Floor
  DATA_IN1 : DataTypeConversion  OutDataTypeStr=boolean  SaturateOnIntegerOverflow=off  RndMeth=Floor
  DATA_IN2 : DataTypeConversion  OutDataTypeStr=boolean  SaturateOnIntegerOverflow=off  RndMeth=Floor
  DATA_IN3 : DataTypeConversion  OutDataTypeStr=boolean  SaturateOnIntegerOverflow=off  RndMeth=Floor
  DATA_IN4 : DataTypeConversion  OutDataTypeStr=inDataType  SaturateOnIntegerOverflow=off  RndMeth=Floor
  HDL Counter : hdlsllib/Sources/HDL Counter  CountType=Count limited  CountInit=0  CountStep=1  CountMax=18800-1  CountFromType=Initial value  CountFrom=0  CountResetPort=off  CountLoadPort=off  CountEnbPort=off  CountDirPort=off  CountHitOutputPort=off  CountDataType=Unsigned  CountWordLen=32  CountFracLen=0  CountSampTime=1/fs
  HDL Counter1 : hdlsllib/Sources/HDL Counter  CountType=Count limited  CountInit=0  CountStep=1  CountMax=1020  CountFromType=Initial value  CountFrom=0  CountResetPort=off  CountLoadPort=off  CountEnbPort=off  CountDirPort=off  CountHitOutputPort=off  CountDataType=Unsigned  CountWordLen=32  CountFracLen=0  CountSampTime=1/fs
  MATLAB Function : MATLAB Function  TreatAsAtomicUnit=on
  simStart : Outport
  simEnd : Outport  Port=2
  simEN : Outport  Port=3
  simDataIn : Outport  Port=4
  wires:
  DATA_IN/1 -> simDataIn/1
  1-D Lookup Table1/1 -> DATA_IN4/1
  HDL Counter1/1 -> 1-D Lookup Table1/1
  DATA_IN3/1 -> simEnd/1
  DATA_IN2/1 -> simStart/1
  DATA_IN1/1 -> simEN/1
  MATLAB Function/3(endSignal) -> DATA_IN3/1
  MATLAB Function/2(start) -> DATA_IN2/1
  MATLAB Function/1(enable) -> DATA_IN1/1
  Constant/1 -> MATLAB Function/1(totalLength)
  HDL Counter/1 -> 1-D Lookup Table/1
  1-D Lookup Table/1 -> DATA_IN/1

== system gm_DVBS/sigSource11 ==
  1-D Lookup Table : Lookup_n-D  NumberOfTableDimensions=1  LookupTableObject=''  BreakpointsForDimension1=[0:18800-1]'  BreakpointsForDimension1FirstPoint=10  BreakpointsForDimension2FirstPoint=10  BreakpointsForDimension1Spacing=12  BreakpointsForDimension2Spacing=12  IndexSearchMethod=Evenly spaced points  Table=sourceData  InterpMethod=Flat  DiagnosticForOutOfRangeInput=Error  InternalRulePriority=Speed  OutDataTypeStr=uint8  RndMeth=Simplest
  1-D Lookup Table1 : Lookup_n-D  Commented=on  NumberOfTableDimensions=1  LookupTableObject=''  BreakpointsForDimension1=[0:1020-1]'  BreakpointsForDimension1FirstPoint=10  BreakpointsForDimension2FirstPoint=10  BreakpointsForDimension1Spacing=12  BreakpointsForDimension2Spacing=12  IndexSearchMethod=Evenly spaced points  Table=oneData  InterpMethod=Flat  DiagnosticForOutOfRangeInput=Error  InternalRulePriority=Speed  OutDataTypeStr=uint8  RndMeth=Simplest
  Constant : Constant  Value=204  OutDataTypeStr=uint16  SampleTime=1/fs
  DATA_IN : DataTypeConversion  OutDataTypeStr=inDataType  SaturateOnIntegerOverflow=off  RndMeth=Floor
  DATA_IN1 : DataTypeConversion  OutDataTypeStr=boolean  SaturateOnIntegerOverflow=off  RndMeth=Floor
  DATA_IN2 : DataTypeConversion  OutDataTypeStr=boolean  SaturateOnIntegerOverflow=off  RndMeth=Floor
  DATA_IN3 : DataTypeConversion  OutDataTypeStr=boolean  SaturateOnIntegerOverflow=off  RndMeth=Floor
  DATA_IN4 : DataTypeConversion  Commented=on  OutDataTypeStr=inDataType  SaturateOnIntegerOverflow=off  RndMeth=Floor
  HDL Counter : hdlsllib/Sources/HDL Counter  CountType=Count limited  CountInit=0  CountStep=1  CountMax=18800-1  CountFromType=Initial value  CountFrom=0  CountResetPort=off  CountLoadPort=off  CountEnbPort=off  CountDirPort=off  CountHitOutputPort=off  CountDataType=Unsigned  CountWordLen=32  CountFracLen=0  CountSampTime=1/fs
  HDL Counter1 : hdlsllib/Sources/HDL Counter  Commented=on  CountType=Count limited  CountInit=0  CountStep=1  CountMax=1020  CountFromType=Initial value  CountFrom=0  CountResetPort=off  CountLoadPort=off  CountEnbPort=off  CountDirPort=off  CountHitOutputPort=off  CountDataType=Unsigned  CountWordLen=32  CountFracLen=0  CountSampTime=1/fs
  MATLAB Function : MATLAB Function  TreatAsAtomicUnit=on
  simStart : Outport
  simEnd : Outport  Port=2
  simEN : Outport  Port=3
  simDataIn : Outport  Port=4
  wires:
  1-D Lookup Table1/1 -> DATA_IN4/1
  HDL Counter1/1 -> 1-D Lookup Table1/1
  DATA_IN3/1 -> simEnd/1
  DATA_IN2/1 -> simStart/1
  DATA_IN1/1 -> simEN/1
  MATLAB Function/3(endSignal) -> DATA_IN3/1
  MATLAB Function/2(start) -> DATA_IN2/1
  MATLAB Function/1(enable) -> DATA_IN1/1
  Constant/1 -> MATLAB Function/1(totalLength)
  DATA_IN/1 -> simDataIn/1
  HDL Counter/1 -> 1-D Lookup Table/1
  1-D Lookup Table/1 -> DATA_IN/1

== system gm_DVBS/Conv_Encoder/int2bin ==
  note: 最低位
  input : Inport
  Demux : Demux  Outputs=8
      settings: DisplayOption=none
  PISO : Subsystem
  Scope3 : Scope  NumInputPorts=4
  Scope4 : Scope  NumInputPorts=4
  uint8tobin : MATLAB Function  TreatAsAtomicUnit=on
  Out1 : Outport
  wires:
  Demux/2 -> Scope3/2, PISO/2(2)
  Demux/3 -> Scope3/3, PISO/3(3)
  Demux/4 -> Scope3/4, PISO/4(4)
  input/1 -> uint8tobin/1(input)
  Demux/7 -> Scope4/3, PISO/7(7)
  Demux/1 -> Scope3/1, PISO/1(1)
  uint8tobin/1(bitValue) -> Demux/1
  Demux/8 -> Scope4/4, PISO/8(8)
  Demux/5 -> Scope4/1, PISO/5(5)
  Demux/6 -> Scope4/2, PISO/6(6)
  PISO/1(Out1) -> Out1/1

== system gm_DVBS/Conv_Encoder/int2bin1 ==
  note: 最低位
  input : Inport
  Demux : Demux  Outputs=8
      settings: DisplayOption=none
  PISO : Subsystem
  Scope3 : Scope  NumInputPorts=4
  Scope4 : Scope  NumInputPorts=4
  uint8tobin : MATLAB Function  TreatAsAtomicUnit=on
  Out1 : Outport
  wires:
  Demux/2 -> Scope3/2, PISO/2(2)
  Demux/3 -> Scope3/3, PISO/3(3)
  Demux/4 -> Scope3/4, PISO/4(4)
  input/1 -> uint8tobin/1(input)
  Demux/7 -> Scope4/3, PISO/7(7)
  Demux/1 -> Scope3/1, PISO/1(1)
  uint8tobin/1(bitValue) -> Demux/1
  Demux/8 -> Scope4/4, PISO/8(8)
  Demux/5 -> Scope4/1, PISO/5(5)
  Demux/6 -> Scope4/2, PISO/6(6)
  PISO/1(Out1) -> Out1/1

== system gm_DVBS/DataSource_Scrambler/CLKdivide ==
  Constant : Constant  Value=8  VectorParams1D=off  OutDataTypeStr=uint8  SampleTime=1/fs
  Constant1 : Constant  Value=25  VectorParams1D=off  OutDataTypeStr=uint8  SampleTime=1/fs
  Delay : Delay  DelayLength=1
  Detect Rise Positive : Subsystem  mask(Detect Rise Positive){vinit=double(0), InputProcessing=Elements as channels (sample based), OutDataTypeStr=boolean}
      mask prompts: vinit "Simulink:masks:InitialCondition_MP"; InputProcessing "Simulink:masks:InputProcessing_MP"; OutDataTypeStr "Simulink:masks:OutputDataType_MP"
      mask help: Simulink:masks:DetectRisePositive_MD
      mask init:
      | InputProcessing = 'Elements as channels (sample based)';
      | OutDataTypeStr = 'boolean';
      | vinit = double(0);
      mask TypeOptions InputProcessing: Simulink:masks:ColumnsAsChannelsFrameBased | Simulink:masks:ElementsAsChannelsSampleBased
      mask TypeOptions OutDataTypeStr: Simulink:masks:uint8 | Simulink:masks:boolean
      mask Display: fprintf('U > 0\n&  NOT\nU/z > 0')
  HDL Counter : hdlsllib/Sources/HDL Counter  CountType=Count limited  CountInit=1  CountStep=1  CountMax=8  CountFromType=Initial value  CountFrom=1  CountResetPort=off  CountLoadPort=off  CountEnbPort=on  CountDirPort=off  CountHitOutputPort=off  CountDataType=Unsigned  CountWordLen=8  CountFracLen=0  CountSampTime=1
  HDL Counter2 : hdlsllib/Sources/HDL Counter  CountType=Count limited  CountInit=1  CountStep=1  CountMax=25  CountFromType=Initial value  CountFrom=1  CountResetPort=off  CountLoadPort=off  CountEnbPort=off  CountDirPort=off  CountHitOutputPort=off  CountDataType=Unsigned  CountWordLen=8  CountFracLen=0  CountSampTime=1/fs
  Relational Operator : RelationalOperator  Operator===  OutDataTypeStr=boolean  InputSameDT=off
  Relational Operator1 : RelationalOperator  Operator===  OutDataTypeStr=boolean  InputSameDT=off
  DataGenEn : Outport  SampleTime=5e-09  VectorParamsAs1DForOutWhenUnconnected=off
  BinEn : Outport  Port=2  SampleTime=5e-09  VectorParamsAs1DForOutWhenUnconnected=off
  wires:
  Constant/1 -> Relational Operator1/2
  Constant1/1 -> Relational Operator/2
  Delay/1 -> BinEn/1
  Detect Rise Positive/1(Y) -> DataGenEn/1
  HDL Counter/1 -> Relational Operator1/1
  HDL Counter2/1 -> Relational Operator/1
  Relational Operator/1 -> Delay/1, HDL Counter/1
  Relational Operator1/1 -> Detect Rise Positive/1(U)

== system gm_DVBS/DataSource_Scrambler/Detect Rise Positive ==
  note: Edge
  note: U(k)
  U : Inport  OutDataTypeStr=boolean  SampleTime=5e-09
  Delay Input1 : UnitDelay  Description=Store in Global RAM  DisableCoverage=on  InitialCondition=vinit  SampleTime=-1  HasFrameUpgradeWarning=on
  FixPt Relational Operator : RelationalOperator  Operator=>  OutDataTypeStr=boolean  ZeroCross=off  InputSameDT=off
  Positive : Subsystem  mask(Compare To Zero){relop=>, OutDataTypeStr=boolean, ZeroCross=off}
      mask prompts: relop "Simulink:masks:Operator_MP"; OutDataTypeStr "Simulink:masks:OutputDataType_MP"; ZeroCross "Simulink:masks:EnableZerocrossingDetection_MP"
      mask help: Simulink:masks:CompareToZero_MD
      mask init:
      | OutDataTypeStr = 'boolean';
      | ZeroCross = 'off';
      | blkName = 'DVBS/DataSource_Scrambler/Detect Rise\nPositive/Positive';
      | relop = '>';
      | setValue = 'boolean';
      mask TypeOptions relop: == | ~= | < | <= | >= | >
      mask TypeOptions OutDataTypeStr: Simulink:masks:uint8 | Simulink:masks:boolean
      mask Callback ZeroCross: sl('zeroCrossEnable', gcbh);
      mask Display: disp([relop,' 0'])
  Y : Outport  SampleTime=5e-09
  wires:
  U/1 -> Positive/1(u)
  Delay Input1/1 -> FixPt Relational Operator/2
  FixPt Relational Operator/1 -> Y/1
  Positive/1(y) -> FixPt Relational Operator/1, Delay Input1/1

== system gm_DVBS/DataSource_Scrambler/Detect Rise Positive1 ==
  note: Edge
  note: U(k)
  U : Inport  OutDataTypeStr=boolean  SampleTime=5e-09
  Delay Input1 : UnitDelay  Description=Store in Global RAM  DisableCoverage=on  InitialCondition=vinit  SampleTime=-1  HasFrameUpgradeWarning=on
  FixPt Relational Operator : RelationalOperator  Operator=>  OutDataTypeStr=boolean  ZeroCross=off  InputSameDT=off
  Positive : Subsystem  mask(Compare To Zero){relop=>, OutDataTypeStr=boolean, ZeroCross=off}
      mask prompts: relop "Simulink:masks:Operator_MP"; OutDataTypeStr "Simulink:masks:OutputDataType_MP"; ZeroCross "Simulink:masks:EnableZerocrossingDetection_MP"
      mask help: Simulink:masks:CompareToZero_MD
      mask init:
      | OutDataTypeStr = 'boolean';
      | ZeroCross = 'off';
      | blkName = 'DVBS/DataSource_Scrambler/Detect Rise\nPositive1/Positive';
      | relop = '>';
      | setValue = 'boolean';
      mask TypeOptions relop: == | ~= | < | <= | >= | >
      mask TypeOptions OutDataTypeStr: Simulink:masks:uint8 | Simulink:masks:boolean
      mask Callback ZeroCross: sl('zeroCrossEnable', gcbh);
      mask Display: disp([relop,' 0'])
  Y : Outport  SampleTime=5e-09
  wires:
  U/1 -> Positive/1(u)
  Delay Input1/1 -> FixPt Relational Operator/2
  FixPt Relational Operator/1 -> Y/1
  Positive/1(y) -> FixPt Relational Operator/1, Delay Input1/1

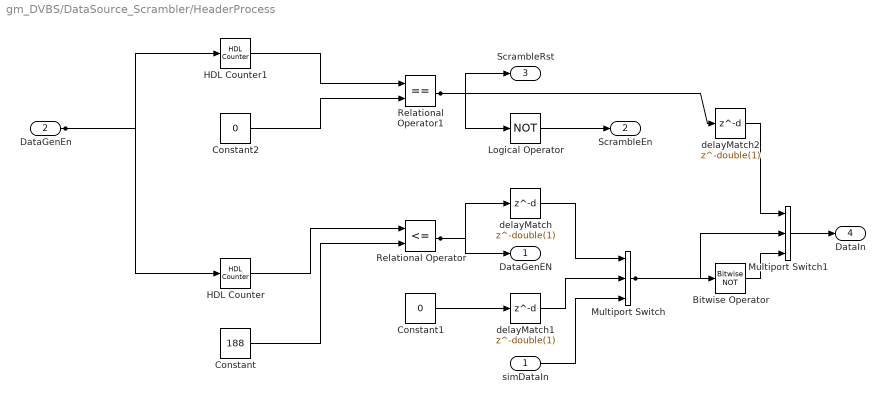
== system gm_DVBS/DataSource_Scrambler/HeaderProcess ==
  simDataIn : Inport  OutDataTypeStr=uint8  PortDimensions=1  SampleTime=5e-09
  DataGenEn : Inport  Port=2  OutDataTypeStr=boolean  PortDimensions=1  SampleTime=5e-09
  Bitwise Operator : simulink/Logic and Bit Operations/Bitwise Operator  logicop=NOT  UseBitMask=off  BitMask=double(0)  BitMaskRealWorld=Real World Value
  Constant : Constant  Value=188  OutDataTypeStr=uint8  SampleTime=5e-09
  Constant1 : Constant  Value=0  OutDataTypeStr=uint8  SampleTime=5e-09
  Constant2 : Constant  Value=0  OutDataTypeStr=uint8  SampleTime=5e-09
  HDL Counter : hdlsllib/Sources/HDL Counter  CountType=Count limited  CountInit=1  CountStep=1  CountMax=n  CountFromType=Initial value  CountFrom=1  CountResetPort=off  CountLoadPort=off  CountEnbPort=on  CountDirPort=off  CountHitOutputPort=off  CountDataType=Unsigned  CountWordLen=8  CountFracLen=0  CountSampTime=1/fs
  HDL Counter1 : hdlsllib/Sources/HDL Counter  CountType=Count limited  CountInit=0  CountStep=1  CountMax=n*8-1  CountFromType=Initial value  CountFrom=0  CountResetPort=off  CountLoadPort=off  CountEnbPort=on  CountDirPort=off  CountHitOutputPort=off  CountDataType=Unsigned  CountWordLen=16  CountFracLen=0  CountSampTime=1/fs
  Logical Operator : Logic  Operator=NOT  Inputs=1  AllPortsSameDT=off  OutDataTypeStr=boolean  SampleTime=5e-09
  Multiport Switch : MultiPortSwitch  DataPortOrder=Specify indices  Inputs=2  DataPortIndices={ double(0) double(1)}  DiagnosticForDefault=None  OutDataTypeStr=uint8  SampleTime=5e-09  SaturateOnIntegerOverflow=off  InputSameDT=off
  Multiport Switch1 : MultiPortSwitch  DataPortOrder=Specify indices  Inputs=2  DataPortIndices={ double(0) double(1)}  DiagnosticForDefault=None  OutDataTypeStr=uint8  SampleTime=5e-09  SaturateOnIntegerOverflow=off  InputSameDT=off
  Relational Operator : RelationalOperator  Operator=<=  OutDataTypeStr=boolean  SampleTime=5e-09  InputSameDT=off
  Relational Operator1 : RelationalOperator  Operator===  OutDataTypeStr=boolean  SampleTime=5e-09  InputSameDT=off
  delayMatch : Delay  DelayLength=double(1)  InitialCondition=0  SampleTime=5e-09
  delayMatch1 : Delay  DelayLength=double(1)  InitialCondition=0  SampleTime=5e-09
  delayMatch2 : Delay  DelayLength=double(1)  InitialCondition=0  SampleTime=5e-09
  DataGenEN : Outport  SampleTime=5e-09  VectorParamsAs1DForOutWhenUnconnected=off
  ScrambleEn : Outport  Port=2  SampleTime=5e-09  VectorParamsAs1DForOutWhenUnconnected=off
  ScrambleRst : Outport  Port=3  SampleTime=5e-09  VectorParamsAs1DForOutWhenUnconnected=off
  DataIn : Outport  Port=4  SampleTime=5e-09
  wires:
  simDataIn/1 -> Multiport Switch/3
  DataGenEn/1 -> HDL Counter/1, HDL Counter1/1
  Bitwise Operator/1 -> Multiport Switch1/3
  Constant/1 -> Relational Operator/2
  delayMatch1/1 -> Multiport Switch/2
  Constant2/1 -> Relational Operator1/2
  HDL Counter/1 -> Relational Operator/1
  HDL Counter1/1 -> Relational Operator1/1
  Logical Operator/1 -> ScrambleEn/1
  Multiport Switch/1 -> Multiport Switch1/2, Bitwise Operator/1
  Multiport Switch1/1 -> DataIn/1
  delayMatch/1 -> Multiport Switch/1
  delayMatch2/1 -> Multiport Switch1/1
  Relational Operator/1 -> delayMatch/1, DataGenEN/1
  Constant1/1 -> delayMatch1/1
  Relational Operator1/1 -> delayMatch2/1, Logical Operator/1, ScrambleRst/1
